simulink model "part2_5"  (R2022a)
settings: Solver=VariableStepAuto  StartTime=0.0  StopTime=10.0  RelTol=1e-3
libraries: dspsnks4 x1
settings Model: Creator=marko  LastModifiedBy=marko
settings SolverCC: MaxZcPerStep=1

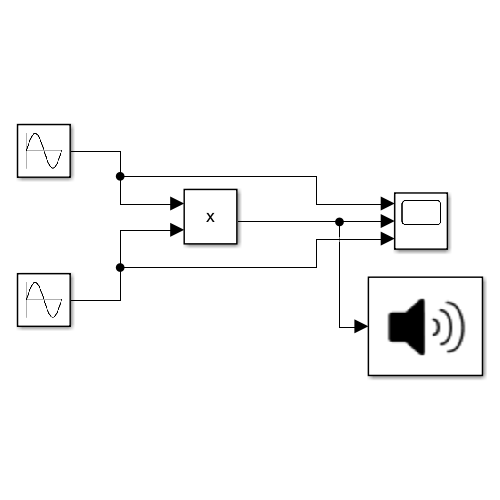
[thumbnail: Simulink's stored preview of the top-level diagram]
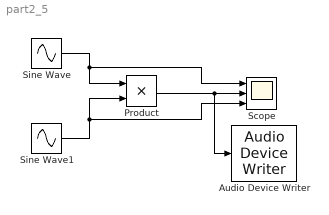
== system part2_5 ==
  Audio Device Writer : dspsnks4/Audio Device Writer  Driver=DirectSound  Device=Default  InheritSampleRate=on  SampleRate=44100  BitDepth=16-bit integer  BufferSize=4096  NumBuffers=10  DefaultOutputChannelMapping=on  OutputChannelMapping=1:2  OutputNumUnderrunSamples=off  DriverIdx=1  DeviceWarnFlag=''
  Product : Product
  Scope : Scope  NumInputPorts=3
  Sine Wave : Sin  Frequency=62.5*pi  SampleTime=0
  Sine Wave1 : Sin  Frequency=1000*pi  SampleTime=0
  wires:
  Sine Wave/1 -> Scope/1, Product/1
  Sine Wave1/1 -> Scope/3, Product/2
  Product/1 -> Scope/2, Audio Device Writer/1
